simulink model "dus4_1"  (R2014a)
settings: Solver=FixedStepDiscrete  StartTime=0.0  StopTime=10.0  FixedStep=0.1  RelTol=1e-3
settings Model: Creator=yoshi12  LastModifiedBy=yoshi12

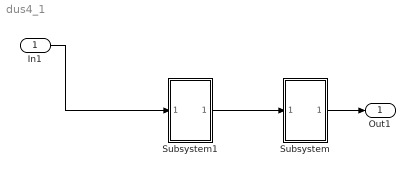
== system dus4_1 ==
  In1 : Inport
  Subsystem : Subsystem
  Subsystem1 : Subsystem
  Out1 : Outport
  wires:
  In1/1 -> Subsystem1/1(In1)
  Subsystem1/1(Out1) -> Subsystem/1(In1)
  Subsystem/1(Out1) -> Out1/1

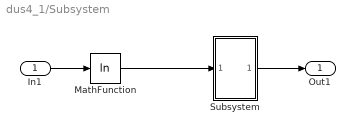
== system dus4_1/Subsystem ==
  In1 : Inport
  MathFunction : Math  Operator=log  SaturateOnIntegerOverflow=on
  Subsystem : Subsystem
  Out1 : Outport
  wires:
  In1/1 -> MathFunction/1
  MathFunction/1 -> Subsystem/1(In1)
  Subsystem/1(Out1) -> Out1/1

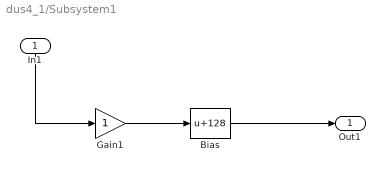
== system dus4_1/Subsystem1 ==
  In1 : Inport
  Bias : Bias  Bias=128
  Gain1 : Gain
  Out1 : Outport
  wires:
  Gain1/1 -> Bias/1
  Bias/1 -> Out1/1
  In1/1 -> Gain1/1

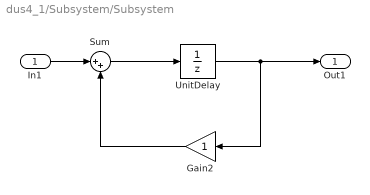
== system dus4_1/Subsystem/Subsystem ==
  In1 : Inport
  Gain2 : Gain
  Sum : Sum  Inputs=|++
  UnitDelay : UnitDelay  SampleTime=-1
  Out1 : Outport
  wires:
  Sum/1 -> UnitDelay/1
  UnitDelay/1 -> Out1/1, Gain2/1
  In1/1 -> Sum/1
  Gain2/1 -> Sum/2
